simulink model "Week1_pr8"  (R2020b)
settings: Solver=VariableStepAuto  StartTime=0.0  StopTime=10.0  RelTol=1e-3
settings Model: Creator=user  LastModifiedBy=user

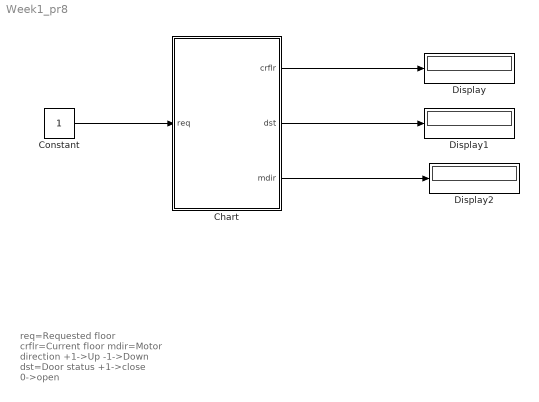
== system Week1_pr8 ==
  note: req=Requested floor
      | crflr=Current floor
      | mdir=Motor direction
      | +1->Up
      | -1->Down
      | dst=Door status
      | +1->close
      | 0->open
  Chart : Stateflow chart  TreatAsAtomicUnit=on
  Constant : Constant
  Display : Display
  Display1 : Display
  Display2 : Display
  wires:
  Chart/1(crflr) -> Display/1
  Chart/3(mdir) -> Display2/1
  Constant/1 -> Chart/1(req)
  Chart/2(dst) -> Display1/1

== stateflow chart Week1_pr8/Chart ==
  state Elevator
    state Idle
      entry:mdir=0;
    state Door_closed
      entry:dst=1;
    state Down
      entry:mdir=-1;
      during:crflr=crflr-1;
    state Up
      entry:mdir=1;
      during:crflr=crflr+1;
    state Stop
      entry:mdir=0;dst=1;
      during:mdir=0;
    state Door_open
      entry:dst=0;
      during:dst=0;mdir=0;
    (default) -> Idle
    Idle -> Idle [order 2] : [req==crflr]
    Door_open -> Idle : after(2,sec)
    Idle -> Door_closed [order 1] : [req~=crflr]
    Door_closed -> Up [order 1] : [req>crflr]
    Door_closed -> Down [order 2] : [req<crflr]
    Down -> Stop : [req==crflr]
    Up -> Stop : [req==crflr]
    Stop -> Door_open : [req==crflr]
  (default) -> Elevator
  data: crflr output =0; req input; dst output; mdir output
